simulink model "ESTS_TFY_test"  (R2023b)
settings: Solver=VariableStepAuto  StartTime=0.0  StopTime=10.0  RelTol=1e-3
libraries: ESTS_TFY x1
settings Model: Creator=blatak  LastModifiedBy=blatak

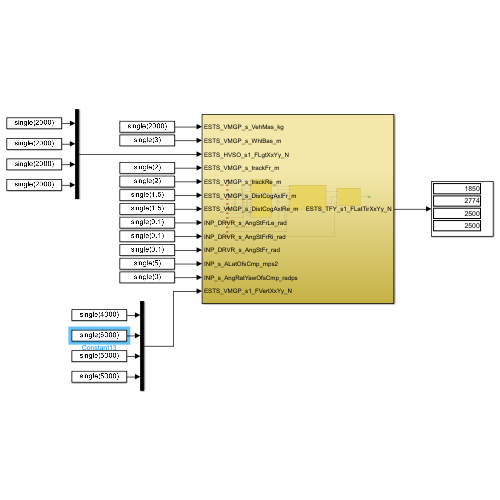
[thumbnail: Simulink's stored preview of the top-level diagram]
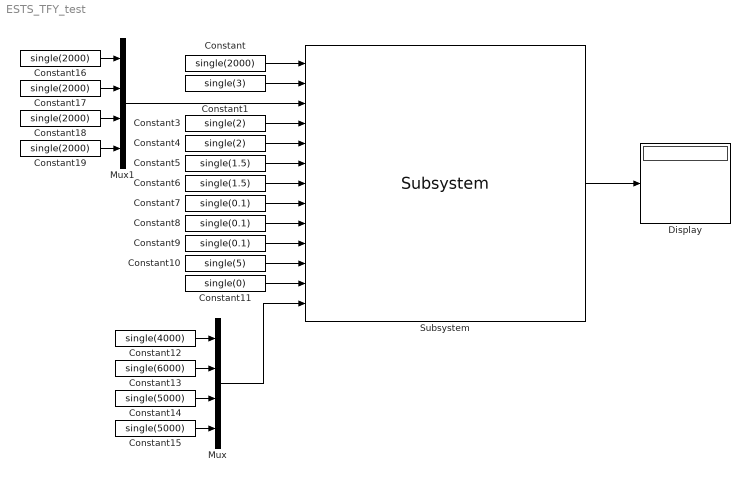
== system ESTS_TFY_test ==
  Constant{,16..19} (5 alike) : Constant  Value=single(2000)
  Constant1 : Constant  Value=single(3)
  Constant10 : Constant  Value=single(5)
  Constant11 : Constant  Value=single(0)
  Constant12 : Constant  Value=single(4000)
  Constant13 : Constant  Value=single(6000)
  Constant14 : Constant  Value=single(5000)
  Constant15 : Constant  Value=single(5000)
  Constant3 : Constant  Value=single(2)
  Constant4 : Constant  Value=single(2)
  Constant5 : Constant  Value=single(1.5)
  Constant6 : Constant  Value=single(1.5)
  Constant7 : Constant  Value=single(0.1)
  Constant8 : Constant  Value=single(0.1)
  Constant9 : Constant  Value=single(0.1)
  Display : Display
  Mux : Mux
  Mux1 : Mux
  Subsystem : ESTS_TFY/Subsystem  SystemSampleTime=-1  VariantActivationTime=update diagram  AllowFlexibleInterface=on  Latency=0  AutoFrameSizeCalculation=off
  wires:
  Constant/1 -> Subsystem/1
  Constant1/1 -> Subsystem/2
  Constant12/1 -> Mux/1
  Constant13/1 -> Mux/2
  Constant14/1 -> Mux/3
  Constant15/1 -> Mux/4
  Mux/1 -> Subsystem/13
  Mux1/1 -> Subsystem/3
  Constant3/1 -> Subsystem/4
  Constant4/1 -> Subsystem/5
  Constant5/1 -> Subsystem/6
  Constant6/1 -> Subsystem/7
  Constant7/1 -> Subsystem/8
  Constant8/1 -> Subsystem/9
  Constant9/1 -> Subsystem/10
  Constant10/1 -> Subsystem/11
  Constant11/1 -> Subsystem/12
  Constant17/1 -> Mux1/2
  Constant19/1 -> Mux1/4
  Constant16/1 -> Mux1/1
  Constant18/1 -> Mux1/3
  Subsystem/1 -> Display/1
